simulink model "untitled"  (R2022a)
settings: Solver=VariableStepAuto  StartTime=0.0  StopTime=20  MaxStep=0.00001  MinStep=0.0000001  RelTol=1e-3
InitFcn:
  | A=[-1 2; 9 0];
  | B=[1;2];
  | C=[6 0];
  | D=-1;
  | L=[0.455; 2.081];
  | K=[-6.6367 4.6833]
settings Model: Creator=Дмитрий  LastModifiedBy=Дмитрий

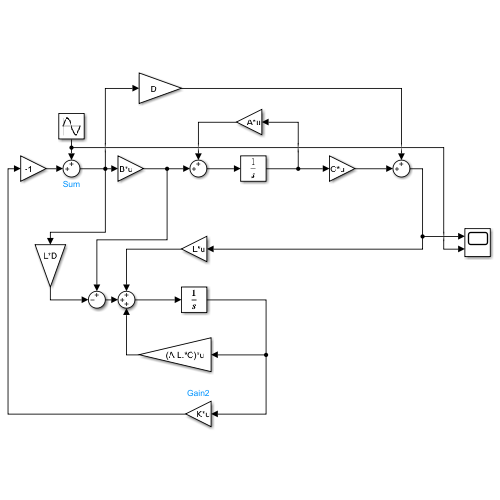
[thumbnail: Simulink's stored preview of the top-level diagram]
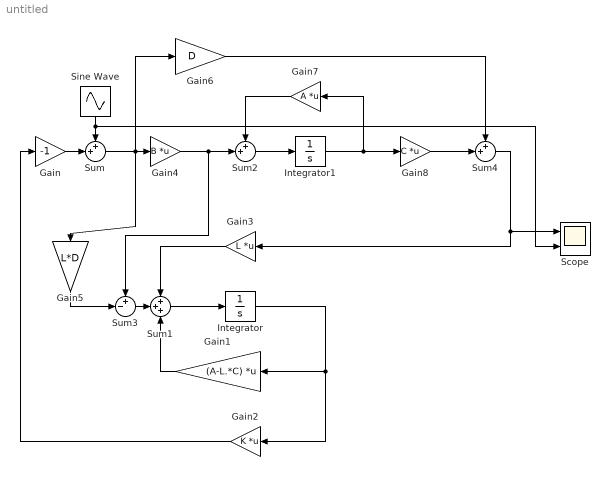
== system untitled ==
  Gain : Gain  Gain=-1
  Gain1 : Gain  Gain=(A-L.*C)  Multiplication=Matrix(K*u)
  Gain2 : Gain  Gain=K  Multiplication=Matrix(K*u)
  Gain3 : Gain  Gain=L  Multiplication=Matrix(K*u)
  Gain4 : Gain  Gain=B  Multiplication=Matrix(K*u)
  Gain5 : Gain  Gain=L*D
  Gain6 : Gain  Gain=D
  Gain7 : Gain  Gain=A  Multiplication=Matrix(K*u)
  Gain8 : Gain  Gain=C  Multiplication=Matrix(K*u)
  Integrator : Integrator
  Integrator1 : Integrator
  Scope : Scope  NumInputPorts=2
  Sine Wave : Sin  Amplitude=2  SampleTime=0
  Sum : Sum  Inputs=++|
  Sum1 : Sum  Inputs=+++
  Sum2 : Sum  Inputs=++|
  Sum3 : Sum  Inputs=+-|
  Sum4 : Sum  Inputs=++|
  wires:
  Sine Wave/1 -> Scope/2, Sum/1
  Gain/1 -> Sum/2
  Sum1/1 -> Integrator/1
  Gain3/1 -> Sum1/1
  Gain1/1 -> Sum1/3
  Integrator/1 -> Gain1/1, Gain2/1
  Sum/1 -> Gain5/1, Gain6/1, Gain4/1
  Gain4/1 -> Sum2/2, Sum3/1
  Gain5/1 -> Sum3/2
  Sum3/1 -> Sum1/2
  Sum2/1 -> Integrator1/1
  Gain7/1 -> Sum2/1
  Integrator1/1 -> Gain7/1, Gain8/1
  Gain8/1 -> Sum4/2
  Gain6/1 -> Sum4/1
  Gain2/1 -> Gain/1
  Sum4/1 -> Gain3/1, Scope/1
